simulink model "PhaseII_opalrt_NoProtection"  (Simulink 8.8)
settings: Solver=ode3  StartTime=0.0  StopTime=inf  FixedStep=Ts  RelTol=1e-5  EnableMultiTasking=on
model workspace (MAT data in the model file):
  Swing_theta = [0 -120 120]
  Swing_v = [1 1 1]
  ft2km = 0.0003048
  miperkm = 0.621371
  w = 376.991118431
  x = 0.5
  x_1 = 10
  x_2 = 1
  x_3 = 1
  x_4 = 1
  x_5 = 1
  x_6 = 1
  x_7 = 1
  x_8 : num (value not decoded)
PostLoadFcn:
  | %BESS ctrl
  | Kpf=0.005*3*12;
  | Kif=5*6;
  | 
  | Kpf1=0.005*3*12;
  | Kif1=5*6;
  | Kp_v=0.016*15*35;
  | Ki_v=12*25;
  | 
  | Kp_v1=0.016*15*35;
  | Ki_v1=12*25;
  | 
  | Vabc_B=12.47e3;
  | Vdc_ref=Vabc_B*2;
  | Kpwm=sqrt(2)*Vabc_B/Vdc_ref;
  | ZB=Vabc_B^2/1e6;
  | R=0.005*ZB;
  | Ibasefull=673/2*sqrt(2);
  | 
  | 
  | Ts_Control=1e-4;
  | ts=0.05;
  | delay=0.2;
  | offset=10e3;
  | t_plan=60;
  | t_monitor=.2;
  | t_mon=t_monitor;
  | scalingfactor=1;
  | x=0.5;
  | n=6;
  | %t_plan=1/15;
  | %t_monitor=10/900;
  | %t_mon=10/900;
  | 
  | %t_plan=1/5;
  | %t_monitor=10/300;
  | %t_mon=10/300;
  | %scalingfactor=1/300;
  | 
  | f0=60;
  | 
  | Pabc_B=1e6;
  | Iabc_B=Pabc_B*sqrt(2/3)/Vabc_B;  % pk value
  | Imax_1=2.5;
  | Ptrans_B=Pabc_B*200;
  | 
  | Vdc_ref=Vabc_B*2;
  | 
  | ZB=Vabc_B^2/Pabc_B;
  | L=0.1*ZB/2/pi/60;
  | R=0.1*ZB;
  | C=1/(4*pi^2*(2e3)^2*L);
  | 
  | LL=0.005*ZB/2/pi/60;
  | RR=0.005*ZB;
  | 
  | RC=0.02;
  | 
  | %%% Initial SOC %%%%
  | SOC_ini_BESS1=0.5;
  | SOC_ini_BESS2=0.5;
  | SOC_ini_BESS3=0.5;
  | 
  | %%% BESS1 %%%
  | fc=200;
  | fc_abc=2e3;
  | 
  | %% Pf droop %%
  | P0_BESS1=0.0*Pabc_B;
  | w0_BESS1=2*pi*60;
  | deltaw=2*pi*0.5;
  | Pmax_BESS1=.1*10;   %% pu value
  | m0_BESS1=deltaw*.5; %deltaw/Pmax_BESS1;    %Pmax_BESS1;
  | kpp_BESS1=3;
  | kpi_BESS1=30;
  | kfp_sec_BESS1=1;
  | kfi_sec_BESS1=30*0.01;
  | Imax_BESS1=Pmax_BESS1;
  | 
  | %% QV droop %%
  | Q0_BESS1=.0*Pabc_B;
  | V0_BESS1=1.03;
  | kvp_BESS1=0.01;
  | kvi_BESS1=5;
  | Dlim=.95;
  | Qmax_BESS1=Pmax_BESS1;
  | mq_BESS1=0.05*.5; %/Qmax_BESS1;
  | kvp_sec_BESS1=1;
  | kvi_sec_BESS1=5*0.05;
  | 
  | %%% BESS2 %%%
  | 
  | %% Pf droop %%
  | P0_BESS2=P0_BESS1;
  | w0_BESS2=2*pi*60;
  | deltaw=2*pi*0.5;
  | Pmax_BESS2=.1*20;   %% pu value
  | m0_BESS2=m0_BESS1;   %/Pmax_BESS2;
  | kpp_BESS2=3;
  | kpi_BESS2=30;
  | Imax_BESS2=Pmax_BESS2;
  | 
  | %% QV droop %%
  | Q0_BESS2=Q0_BESS1;
  | V0_BESS2=V0_BESS1;
  | kvp_BESS2=0.01;
  | kvi_BESS2=5;
  | Qmax_BESS2=Pmax_BESS2;
  | mq_BESS2=mq_BESS1;   %/Qmax_BESS2;
  | 
  | %%% BESS3 %%%
  | 
  | %% Pf droop %%
  | P0_BESS3=0.0*Pabc_B;
  | w0_BESS3=2*pi*60;
  | deltaw=2*pi*0.5;
  | Pmax_BESS3=.1*6;   %% pu value
  | m0_BESS3=deltaw*.5; %deltaw/Pmax_BESS3;    %Pmax_BESS1;
  | kpp_BESS3=3;
  | kpi_BESS3=30;
  | kfp_sec_BESS3=1;
  | kfi_sec_BESS3=30*0.01;
  | Imax_BESS3=Pmax_BESS3;
  | 
  | %% QV droop %%
  | Q0_BESS3=.0*Pabc_B;
  | V0_BESS3=1.03;
  | kvp_BESS3=0.01;
  | kvi_BESS3=5;
  | Dlim=.95;
  | Qmax_BESS3=Pmax_BESS3;
  | mq_BESS3=0.05*.5; %/Qmax_BESS3;
  | kvp_sec_BESS3=1;
  | kvi_sec_BESS3=5*0.05;
  | 
  | 
  | %% Outer voltage and inner current loops %%%
  | %Kp_v=0.19*0.036*20;
  | %Ki_v=0.19*5;
  | 
  | % Kp_I=2.773*0.0013/10/1.5;
  | % Ki_I =2.773/5/1.5;
  | Kp_I=2.773*0.0013; %ma /2phil 0413 /2
  | Ki_I =2.773/2/1.5; %ma /2phil 0413 /2
  | 
  | 
  | % Kp_I_PV=2.773*0.0013/2/500;
  | % Ki_I_PV =2.773/1/20000;
  | % Kp_I_PV=2.773*0.0013/10/1.5;
  | % Ki_I_PV =2.773/5/1.5;
  | Kp_I_PV=2.773*0.0013/4; %ma /2phil 0413 /2
  | Ki_I_PV =2.773/2/1.5/4; %ma /2phil 0413 /2
  | 
  | %%% single voltage loop %%%
  | Kp_vd=0.053*0.0042*0.02;
  | Ki_vd=0.053*0.02;
  | 
  | Kp_vd_neg=0.053*0.0042*0.1;
  | Ki_vd_neg=0.053*0.1;
  | 
  | coupling_pu=w0_BESS1*L/ZB*Vabc_B/Vdc_ref*1.414;%*sqrt(2)
  | 
  | 
  | %%% Load %%%
  | 
  | %% Critical Load %%
  | Pref_CL1=-161e3;
  | Qref_CL1=-50e3*0;
  | 
  | Pref_CL2=-161e3;
  | Qref_CL2=-50e3*0;
  | 
  | %% Non-critical load %%
  | Pref_NCL=-505e3*1;
  | Qref_NCL=-50e3*0;
  | 
  | %%% PV %%%
  | Qref_PV1=100e3*0;
  | Qref_PV2=100e3*0;
  | 
  | %%% BESS1 %%%
  | Pref_BESS1=100e3;
  | Qref_BESS1=100e3;
  | 
  | %%% BESS2 %%%
  | Pref_BESS2=500e3;
  | Qref_BESS2=500e3;
  | 
  | %%% Islanded detection %%%%
  | kneg=0.01;
  | Vneg_trip=0.04;
  | Nhit=50;
  | Kp_I_neg=2.773*0.0013/8;
  | Ki_I_neg =2.773/8;
  | 
  | %%% Resynchronization %%%%
  | kp_theta_BESS1=kpp_BESS1*3*10;
  | ki_theta_BESS1=kpi_BESS1*1*10;
  | kp_theta_BESS2=kp_theta_BESS1;
  | ki_theta_BESS2=ki_theta_BESS1;
  | 
  | kvp_resyn_BESS1=kvp_BESS1*3;
  | kvi_resyn_BESS1=kvi_BESS1*3;
  | kvp_resyn_BESS2=kvp_resyn_BESS1;
  | kvi_resyn_BESS2=kvi_resyn_BESS1;
  | 
  | %%% Virtual Impedance %%%%
  | L_vir=4.6685e-3;
  | R_vir=0;
  | 
  | %% harmonic compensation %%%%
  | Smax_BESS1=0.5;
  | Smax_BESS2=0.5;
  | Rvir_BESS1=-1*1;
  | Rvir_BESS2=Rvir_BESS1/1.5;
  | Lvir_BESS1=-40e-3;
  | Lvir_BESS2=Lvir_BESS1/1.5;
  | 
  | t_resyn=.25*10;
  | topen=.45*10;
  | tfault=20;
  | t_run=0.15*10;
  | Imax_BESS3_ini=3;
  | 
  | td_trans=1*1/f0;
  | td_comm=10e-3*1; Ts = 1e-4;
  | 
  | PV_0 = [0,0,0,0,0,0,0,0,0,0,0,0,0,0,0,0,0,0,0,0,0,0,0,0.00637590701003014,0.0597883305113194,0.191640198758314,0.258183655928258,0.318938480096502,0.451835046830676,0.659184087530387,0.827159209540989,1.02022332643508,1.18871489543793,1.35005293581671,1.44694872050258,1.52351715157350,1.70617264822951,1.84211772778079,1.88159346030552,1.92819173463478,1.95215782620083,1.94381351836891,2,1.97817052341903,1.98389128053032,1.95943530210305,1.90454584020392,1.83270216133066,1.74331256478643,1.68711132752699,1.64586049291177,1.53600483984610,1.40476385461279,1.29483442340538,1.11929409073974,0.908933426293792,0.676474732830904,0.512353780945319,0.359824850691486,0.238560145785608,0.135084826418477,0.0524857700409100,0.00608374556870036,0,0,0,0,0,0,0,0,0,0,0,0,0,0,0,0,0,0,0,0,0,0,0,0,0,0,0,0,0,0];
  | BESS_limit=1.5;
  | 
  | 
  | B_OL = [6.9443e-06 2.8805e-06];
  | B_UG = [6.00927e-05 3.73399e-05];
  | Omega = 376.9911184307752;
  | R_OL = [0.17 0.527];
  | R_UG = [0.1853 0.8313];
  | X_OL = [0.6283 2.0185];
  | X_UG = [0.3144 0.3404];
  | ft2km = 0.0003048;
  | load_scale = 0.5;
  | 
  | 
  | wb = 2*pi*60; %frequency of input voltage
  | Vb = 12.47e3*sqrt(2/3); % phase voltage amplitude
  | Pb = 1e6; % Pb=2.552kW
  | Ib = Pb/(3/2*Vb); %pha
  | %%generator electrical parameters, stator resistance ignored
  | xd=3.4375;
  | xq=1.7499;
  | xdp=0.2626;
  | xqp=0.1790;
  | Td0p=2.389;
  | Tq0p=0.07;
  | 
  | %%excitation
  | KA=200;
  | TA=0.01;
  | Efdmin=-4.5; %% field voltage lower limit
  | Efdmax=4.5; %% field voltage upper limit
  | 
  | %%inertia
  | H1=7;%6.5;
  | H2=10;%6.175;
  | D=2;
  | M1=2*H1;
  | M2=2*H2;
  | 
  | %%AGC parameters (different parameters in the simulation; AGC integrates every 2 seconds, disabled before 70s)
  | B1=41; %%in simulation B1=21
  | KI=0.8; %%in simulation KI=0.05
  | 
  | %%droop
  | R_1=20;
  | 
  | %%governor
  | TG=0.2;
  | 
  | %%turbine
  | FHP=0.3;
  | TRH=7.0;
  | TCH=0.3;
  | 
  | Ts=8e-5;
InitFcn:
  | %BESS ctrl
  | Kpf=0.005*3*12;
  | Kif=5*6;
  | 
  | Kpf1=0.005*3*12;
  | Kif1=5*6;
  | Kp_v=0.016*15*35;
  | Ki_v=12*25;
  | 
  | Kp_v1=0.016*15*35;
  | Ki_v1=12*25;
  | 
  | Vabc_B=12.47e3;
  | Vdc_ref=Vabc_B*2;
  | Kpwm=sqrt(2)*Vabc_B/Vdc_ref;
  | ZB=Vabc_B^2/1e6;
  | R=0.005*ZB;
  | Ibasefull=673/2*sqrt(2);
  | 
  | 
  | Ts_Control=1e-4;
  | ts=0.05;
  | delay=0.2;
  | offset=10e3;
  | t_plan=60;
  | t_monitor=.2;
  | t_mon=t_monitor;
  | scalingfactor=1;
  | x=0.5;
  | n=6;
  | %t_plan=1/15;
  | %t_monitor=10/900;
  | %t_mon=10/900;
  | 
  | %t_plan=1/5;
  | %t_monitor=10/300;
  | %t_mon=10/300;
  | %scalingfactor=1/300;
  | 
  | f0=60;
  | 
  | Pabc_B=1e6;
  | Iabc_B=Pabc_B*sqrt(2/3)/Vabc_B;  % pk value
  | Imax_1=2.5;
  | Ptrans_B=Pabc_B*200;
  | 
  | Vdc_ref=Vabc_B*2;
  | 
  | ZB=Vabc_B^2/Pabc_B;
  | L=0.1*ZB/2/pi/60;
  | R=0.1*ZB;
  | C=1/(4*pi^2*(2e3)^2*L);
  | 
  | LL=0.005*ZB/2/pi/60;
  | RR=0.005*ZB;
  | 
  | RC=0.02;
  | 
  | %%% Initial SOC %%%%
  | SOC_ini_BESS1=0.5;
  | SOC_ini_BESS2=0.5;
  | SOC_ini_BESS3=0.5;
  | 
  | %%% BESS1 %%%
  | fc=200;
  | fc_abc=2e3;
  | 
  | %% Pf droop %%
  | P0_BESS1=0.0*Pabc_B;
  | w0_BESS1=2*pi*60;
  | deltaw=2*pi*0.5;
  | Pmax_BESS1=.1*10;   %% pu value
  | m0_BESS1=deltaw*.5; %deltaw/Pmax_BESS1;    %Pmax_BESS1;
  | kpp_BESS1=3;
  | kpi_BESS1=30;
  | kfp_sec_BESS1=1;
  | kfi_sec_BESS1=30*0.01;
  | Imax_BESS1=Pmax_BESS1;
  | 
  | %% QV droop %%
  | Q0_BESS1=.0*Pabc_B;
  | V0_BESS1=1.03;
  | kvp_BESS1=0.01;
  | kvi_BESS1=5;
  | Dlim=.95;
  | Qmax_BESS1=Pmax_BESS1;
  | mq_BESS1=0.05*.5; %/Qmax_BESS1;
  | kvp_sec_BESS1=1;
  | kvi_sec_BESS1=5*0.05;
  | 
  | %%% BESS2 %%%
  | 
  | %% Pf droop %%
  | P0_BESS2=P0_BESS1;
  | w0_BESS2=2*pi*60;
  | deltaw=2*pi*0.5;
  | Pmax_BESS2=.1*20;   %% pu value
  | m0_BESS2=m0_BESS1;   %/Pmax_BESS2;
  | kpp_BESS2=3;
  | kpi_BESS2=30;
  | Imax_BESS2=Pmax_BESS2;
  | 
  | %% QV droop %%
  | Q0_BESS2=Q0_BESS1;
  | V0_BESS2=V0_BESS1;
  | kvp_BESS2=0.01;
  | kvi_BESS2=5;
  | Qmax_BESS2=Pmax_BESS2;
  | mq_BESS2=mq_BESS1;   %/Qmax_BESS2;
  | 
  | %%% BESS3 %%%
  | 
  | %% Pf droop %%
  | P0_BESS3=0.0*Pabc_B;
  | w0_BESS3=2*pi*60;
  | deltaw=2*pi*0.5;
  | Pmax_BESS3=.1*6;   %% pu value
  | m0_BESS3=deltaw*.5; %deltaw/Pmax_BESS3;    %Pmax_BESS1;
  | kpp_BESS3=3;
  | kpi_BESS3=30;
  | kfp_sec_BESS3=1;
  | kfi_sec_BESS3=30*0.01;
  | Imax_BESS3=Pmax_BESS3;
  | 
  | %% QV droop %%
  | Q0_BESS3=.0*Pabc_B;
  | V0_BESS3=1.03;
  | kvp_BESS3=0.01;
  | kvi_BESS3=5;
  | Dlim=.95;
  | Qmax_BESS3=Pmax_BESS3;
  | mq_BESS3=0.05*.5; %/Qmax_BESS3;
  | kvp_sec_BESS3=1;
  | kvi_sec_BESS3=5*0.05;
  | 
  | 
  | %% Outer voltage and inner current loops %%%
  | %Kp_v=0.19*0.036*20;
  | %Ki_v=0.19*5;
  | 
  | % Kp_I=2.773*0.0013/10/1.5;
  | % Ki_I =2.773/5/1.5;
  | Kp_I=2.773*0.0013; %ma /2phil 0413 /2
  | Ki_I =2.773/2/1.5; %ma /2phil 0413 /2
  | 
  | 
  | % Kp_I_PV=2.773*0.0013/2/500;
  | % Ki_I_PV =2.773/1/20000;
  | % Kp_I_PV=2.773*0.0013/10/1.5;
  | % Ki_I_PV =2.773/5/1.5;
  | Kp_I_PV=2.773*0.0013/4; %ma /2phil 0413 /2
  | Ki_I_PV =2.773/2/1.5/4; %ma /2phil 0413 /2
  | 
  | %%% single voltage loop %%%
  | Kp_vd=0.053*0.0042*0.02;
  | Ki_vd=0.053*0.02;
  | 
  | Kp_vd_neg=0.053*0.0042*0.1;
  | Ki_vd_neg=0.053*0.1;
  | 
  | coupling_pu=w0_BESS1*L/ZB*Vabc_B/Vdc_ref*1.414;%*sqrt(2)
  | 
  | 
  | %%% Load %%%
  | 
  | %% Critical Load %%
  | Pref_CL1=-161e3;
  | Qref_CL1=-50e3*0;
  | 
  | Pref_CL2=-161e3;
  | Qref_CL2=-50e3*0;
  | 
  | %% Non-critical load %%
  | Pref_NCL=-505e3*1;
  | Qref_NCL=-50e3*0;
  | 
  | %%% PV %%%
  | Qref_PV1=100e3*0;
  | Qref_PV2=100e3*0;
  | 
  | %%% BESS1 %%%
  | Pref_BESS1=100e3;
  | Qref_BESS1=100e3;
  | 
  | %%% BESS2 %%%
  | Pref_BESS2=500e3;
  | Qref_BESS2=500e3;
  | 
  | %%% Islanded detection %%%%
  | kneg=0.01;
  | Vneg_trip=0.04;
  | Nhit=50;
  | Kp_I_neg=2.773*0.0013/8;
  | Ki_I_neg =2.773/8;
  | 
  | %%% Resynchronization %%%%
  | kp_theta_BESS1=kpp_BESS1*3*10;
  | ki_theta_BESS1=kpi_BESS1*1*10;
  | kp_theta_BESS2=kp_theta_BESS1;
  | ki_theta_BESS2=ki_theta_BESS1;
  | 
  | kvp_resyn_BESS1=kvp_BESS1*3;
  | kvi_resyn_BESS1=kvi_BESS1*3;
  | kvp_resyn_BESS2=kvp_resyn_BESS1;
  | kvi_resyn_BESS2=kvi_resyn_BESS1;
  | 
  | %%% Virtual Impedance %%%%
  | L_vir=4.6685e-3;
  | R_vir=0;
  | 
  | %% harmonic compensation %%%%
  | Smax_BESS1=0.5;
  | Smax_BESS2=0.5;
  | Rvir_BESS1=-1*1;
  | Rvir_BESS2=Rvir_BESS1/1.5;
  | Lvir_BESS1=-40e-3;
  | Lvir_BESS2=Lvir_BESS1/1.5;
  | 
  | t_resyn=.25*10;
  | topen=.45*10;
  | tfault=20;
  | t_run=0.15*10;
  | Imax_BESS3_ini=3;
  | 
  | td_trans=1*1/f0;
  | td_comm=10e-3*1; Ts = 1e-4;
  | 
  | PV_0 = [0,0,0,0,0,0,0,0,0,0,0,0,0,0,0,0,0,0,0,0,0,0,0,0.00637590701003014,0.0597883305113194,0.191640198758314,0.258183655928258,0.318938480096502,0.451835046830676,0.659184087530387,0.827159209540989,1.02022332643508,1.18871489543793,1.35005293581671,1.44694872050258,1.52351715157350,1.70617264822951,1.84211772778079,1.88159346030552,1.92819173463478,1.95215782620083,1.94381351836891,2,1.97817052341903,1.98389128053032,1.95943530210305,1.90454584020392,1.83270216133066,1.74331256478643,1.68711132752699,1.64586049291177,1.53600483984610,1.40476385461279,1.29483442340538,1.11929409073974,0.908933426293792,0.676474732830904,0.512353780945319,0.359824850691486,0.238560145785608,0.135084826418477,0.0524857700409100,0.00608374556870036,0,0,0,0,0,0,0,0,0,0,0,0,0,0,0,0,0,0,0,0,0,0,0,0,0,0,0,0,0,0];
  | BESS_limit=1.5;
  | 
  | 
  | B_OL = [6.9443e-06 2.8805e-06];
  | B_UG = [6.00927e-05 3.73399e-05];
  | Omega = 376.9911184307752;
  | R_OL = [0.17 0.527];
  | R_UG = [0.1853 0.8313];
  | X_OL = [0.6283 2.0185];
  | X_UG = [0.3144 0.3404];
  | ft2km = 0.0003048;
  | load_scale = 0.5;
  | 
  | 
  | wb = 2*pi*60; %frequency of input voltage
  | Vb = 12.47e3*sqrt(2/3); % phase voltage amplitude
  | Pb = 1e6; % Pb=2.552kW
  | Ib = Pb/(3/2*Vb); %pha
  | %%generator electrical parameters, stator resistance ignored
  | xd=3.4375;
  | xq=1.7499;
  | xdp=0.2626;
  | xqp=0.1790;
  | Td0p=2.389;
  | Tq0p=0.07;
  | 
  | %%excitation
  | KA=200;
  | TA=0.01;
  | Efdmin=-4.5; %% field voltage lower limit
  | Efdmax=4.5; %% field voltage upper limit
  | 
  | %%inertia
  | H1=7;%6.5;
  | H2=10;%6.175;
  | D=2;
  | M1=2*H1;
  | M2=2*H2;
  | 
  | %%AGC parameters (different parameters in the simulation; AGC integrates every 2 seconds, disabled before 70s)
  | B1=41; %%in simulation B1=21
  | KI=0.8; %%in simulation KI=0.05
  | 
  | %%droop
  | R_1=20;
  | 
  | %%governor
  | TG=0.2;
  | 
  | %%turbine
  | FHP=0.3;
  | TRH=7.0;
  | TCH=0.3;
  | 
  | Ts=8e-5;
undefined symbols (not defined in the file): D1, Delta, DiscIntNeverNeededParam, Left, PG2ref, type, V
libraries: powerlib x220, powerlib_meascontrol x82, dspstat3 x54, dsparch4 x43, dspswit3 x24, simulink x19, simulink_extras x12, powerlib_extras x11, ssn_lib x7, artemis x6, rtlab x5, rtio_generic_dnp3 x5
(part 1 of 9)
settings Model: ARTEMISmethode_block_infos=$$__separator__$$PhaseII_opalrt_NoProtection/ARTEMIS Guide$$__separator__$$  Creator=AmineYamane  LastModifiedBy=iray1
settings OptimizationCC: BlockReduction=off  BooleanDataType=off  OptimizeBlockIOStorage=off  BufferReuse=off  GlobalBufferReuse=off  ExpressionFolding=off  ExpressionDepthLimit=2147483647  LocalBlockOutputs=off
settings DebuggingCC: SolverPrmCheckMsg=warning  MultiTaskCondExecSysMsg=warning  UnconnectedInputMsg=none  UnconnectedOutputMsg=none  UnconnectedLineMsg=none
settings ModelReferenceCC: ModelReferenceMinAlgLoopOccurrences=on
settings ConfigComp: CovSFcnEnable=off

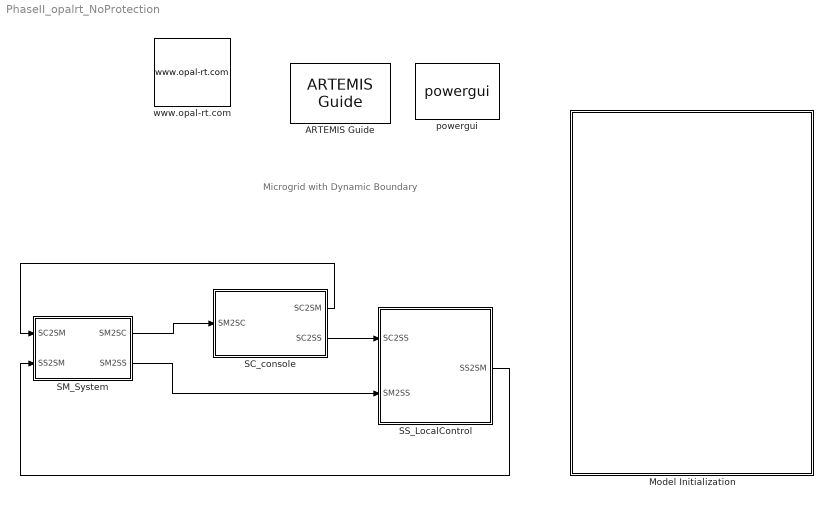
== system PhaseII_opalrt_NoProtection ==
  note: Microgrid with Dynamic Boundary
  ARTEMIS Guide : artemis/ARTEMIS/ARTEMIS Guide  Tag=FTSSmethode_opal_4hx0r99  Description=5.0_z1  lock=on  Ts=Ts  opt=art5  dyna=off  nb_perm=50  RT_fullcomp=off  ssn=on  ssn_itvc=off  ssn_ivic=off  ssn_ext=off  ssn_solver=Backward Euler  ssn_impulse=off  ssn_quasimpulse=off  ssn_impulse_loop=2  paraExtinctionThy=off  Thy_Impulse=on  dtc=Off  dtc_opt=true impulse event detection  ao=on  simtype=off  ct_mac=off  lin_mov=off  lsp=[0.001 2]  spike_skip=Disabled  dtc_extra=1  dtc_sws=normal  dtc_pied=0.5  SPSRulesBlock=SPSRules  tre=on  ctmm=off  LF=off  dpl_type=ARTEMiS DPL  rlc_type=off  custom_type=off  para=off  ssn_ImpulseLoopBlockedStateUpdate=2  ssn_mov_iter_number=5  ssn_switch_iter_number=5  ssn_nib_type_verify=on  ssn_use_lu=on  ssn_use_ldlt=off
  Model Initialization : Subsystem  mask(Model Functions){InitFcnX=|, prel=off, posl=on, inif=on, strf=off}
      mask InitFcnX=|
      | %BESS ctrl
      | Kpf=0.005*3*12;
      | Kif=5*6;
      |
      | Kpf1=0.005*3*12;
      | Kif1=5*6;
      | Kp_v=0.016*15*35;
      | Ki_v=12*25;
      |
      | Kp_v1=0.016*15*35;
      | Ki_v1=12*25;
      |
      | Vabc_B=12.47e3;
      | Vdc_ref=Vabc_B*2;
      | Kpwm=sqrt(2)*Vabc_B/Vdc_ref;
      | ZB=Vabc_B^2/1e6;
      | R=0.005*ZB;
      | Ibasefull=673/2*sqrt(2);
      |
      |
      | Ts_Control=1e-4;
      | ts=0.05;
      | delay=0.2;
      | offset=10e3;
      | t_plan=60;
      | t_monitor=.2;
      | t_mon=t_monitor;
      | scalingfactor=1;
      | x=0.5;
      | n=6;
      | %t_plan=1/15;
      | %t_monitor=10/900;
      | %t_mon=10/900;
      |
      | %t_plan=1/5;
      | %t_monitor=10/300;
      | %t_mon=10/300;
      | %scalingfactor=1/300;
      |
      | f0=60;
      |
      | Pabc_B=1e6;
      | Iabc_B=Pabc_B*sqrt(2/3)/Vabc_B;  % pk value
      | Imax_1=2.5;
      | Ptrans_B=Pabc_B*200;
      |
      | Vdc_ref=Vabc_B*2;
      |
      | ZB=Vabc_B^2/Pabc_B;
      | L=0.1*ZB/2/pi/60;
      | R=0.1*ZB;
      | C=1/(4*pi^2*(2e3)^2*L);
      |
      | LL=0.005*ZB/2/pi/60;
      | RR=0.005*ZB;
      |
      | RC=0.02;
      |
      | %%% Initial SOC %%%%
      | SOC_ini_BESS1=0.5;
      | SOC_ini_BESS2=0.5;
      | SOC_ini_BESS3=0.5;
      |
      | %%% BESS1 %%%
      | fc=200;
      | fc_abc=2e3;
      |
      | %% Pf droop %%
      | P0_BESS1=0.0*Pabc_B;
      | w0_BESS1=2*pi*60;
      | deltaw=2*pi*0.5;
      | Pmax_BESS1=.1*10;   %% pu value
      | m0_BESS1=deltaw*.5; %deltaw/Pmax_BESS1;    %Pmax_BESS1;
      | kpp_BESS1=3;
      | kpi_BESS1=30;
      | kfp_sec_BESS1=1;
      | kfi_sec_BESS1=30*0.01;
      | Imax_BESS1=Pmax_BESS1;
      |
      | %% QV droop %%
      | Q0_BESS1=.0*Pabc_B;
      | V0_BESS1=1.03;
      | kvp_BESS1=0.01;
      | kvi_BESS1=5;
      | Dlim=.95;
      | Qmax_BESS1=Pmax_BESS1;
      | mq_BESS1=0.05*.5; %/Qmax_BESS1;
      | kvp_sec_BESS1=1;
      | kvi_sec_BESS1=5*0.05;
      |
      | %%% BESS2 %%%
      |
      | %% Pf droop %%
      | P0_BESS2=P0_BESS1;
      | w0_BESS2=2*pi*60;
      | deltaw=2*pi*0.5;
      | Pmax_BESS2=.1*20;   %% pu value
      | m0_BESS2=m0_BESS1;   %/Pmax_BESS2;
      | kpp_BESS2=3;
      | kpi_BESS2=30;
      | Imax_BESS2=Pmax_BESS2;
      |
      | %% QV droop %%
      | Q0_BESS2=Q0_BESS1;
      | V0_BESS2=V0_BESS1;
      | kvp_BESS2=0.01;
      | kvi_BESS2=5;
      | Qmax_BESS2=Pmax_BESS2;
      | mq_BESS2=mq_BESS1;   %/Qmax_BESS2;
      |
      | %%% BESS3 %%%
      |
      | %% Pf droop %%
      | P0_BESS3=0.0*Pabc_B;
      | w0_BESS3=2*pi*60;
      | deltaw=2*pi*0.5;
      | Pmax_BESS3=.1*6;   %% pu value
      | m0_BESS3=deltaw*.5; %deltaw/Pmax_BESS3;    %Pmax_BESS1;
      | kpp_BESS3=3;
      | kpi_BESS3=30;
      | kfp_sec_BESS3=1;
      | kfi_sec_BESS3=30*0.01;
      | Imax_BESS3=Pmax_BESS3;
      |
      | %% QV droop %%
      | Q0_BESS3=.0*Pabc_B;
      | V0_BESS3=1.03;
      | kvp_BESS3=0.01;
      | kvi_BESS3=5;
      | Dlim=.95;
      | Qmax_BESS3=Pmax_BESS3;
      | mq_BESS3=0.05*.5; %/Qmax_BESS3;
      | kvp_sec_BESS3=1;
      | kvi_sec_BESS3=5*0.05;
      |
      |
      | %% Outer voltage and inner current loops %%%
      | %Kp_v=0.19*0.036*20;
      | %Ki_v=0.19*5;
      |
      | % Kp_I=2.773*0.0013/10/1.5;
      | % Ki_I =2.773/5/1.5;
      | Kp_I=2.773*0.0013; %ma /2phil 0413 /2
      | Ki_I =2.773/2/1.5; %ma /2phil 0413 /2
      |
      |
      | % Kp_I_PV=2.773*0.0013/2/500;
      | % Ki_I_PV =2.773/1/20000;
      | % Kp_I_PV=2.773*0.0013/10/1.5;
      | % Ki_I_PV =2.773/5/1.5;
      | Kp_I_PV=2.773*0.0013/4; %ma /2phil 0413 /2
      | Ki_I_PV =2.773/2/1.5/4; %ma /2phil 0413 /2
      |
      | %%% single voltage loop %%%
      | Kp_vd=0.053*0.0042*0.02;
      | Ki_vd=0.053*0.02;
      |
      | Kp_vd_neg=0.053*0.0042*0.1;
      | Ki_vd_neg=0.053*0.1;
      |
      | coupling_pu=w0_BESS1*L/ZB*Vabc_B/Vdc_ref*1.414;%*sqrt(2)
      |
      |
      | %%% Load %%%
      |
      | %% Critical Load %%
      | Pref_CL1=-161e3;
      | Qref_CL1=-50e3*0;
      |
      | Pref_CL2=-161e3;
      | Qref_CL2=-50e3*0;
      |
      | %% Non-critical load %%
      | Pref_NCL=-505e3*1;
      | Qref_NCL=-50e3*0;
      |
      | %%% PV %%%
      | Qref_PV1=100e3*0;
      | Qref_PV2=100e3*0;
      |
      | %%% BESS1 %%%
      | Pref_BESS1=100e3;
      | Qref_BESS1=100e3;
      |
      | %%% BESS2 %%%
      | Pref_BESS2=500e3;
      | Qref_BESS2=500e3;
      |
      | %%% Islanded detection %%%%
      | kneg=0.01;
      | Vneg_trip=0.04;
      | Nhit=50;
      | Kp_I_neg=2.773*0.0013/8;
      | Ki_I_neg =2.773/8;
      |
      | %%% Resynchronization %%%%
      | kp_theta_BESS1=kpp_BESS1*3*10;
      | ki_theta_BESS1=kpi_BESS1*1*10;
      | kp_theta_BESS2=kp_theta_BESS1;
      | ki_theta_BESS2=ki_theta_BESS1;
      |
      | kvp_resyn_BESS1=kvp_BESS1*3;
      | kvi_resyn_BESS1=kvi_BESS1*3;
      | kvp_resyn_BESS2=kvp_resyn_BESS1;
      | kvi_resyn_BESS2=kvi_resyn_BESS1;
      |
      | %%% Virtual Impedance %%%%
      | L_vir=4.6685e-3;
      | R_vir=0;
      |
      | %% harmonic compensation %%%%
      | Smax_BESS1=0.5;
      | Smax_BESS2=0.5;
      | Rvir_BESS1=-1*1;
      | Rvir_BESS2=Rvir_BESS1/1.5;
      | Lvir_BESS1=-40e-3;
      | Lvir_BESS2=Lvir_BESS1/1.5;
      |
      | t_resyn=.25*10;
      | topen=.45*10;
      | tfault=20;
      | t_run=0.15*10;
      | Imax_BESS3_ini=3;
      |
      | td_trans=1*1/f0;
      | td_comm=10e-3*1; Ts = 1e-4;
      |
      | PV_0 = [0,0,0,0,0,0,0,0,0,0,0,0,0,0,0,0,0,0,0,0,0,0,0,0.00637590701003014,0.0597883305113194,0.191640198758314,0.258183655928258,0.318938480096502,0.451835046830676,0.659184087530387,0.827159209540989,1.02022332643508,1.18871489543793,1.35005293581671,1.44694872050258,1.52351715157350,1.70617264822951,1.84211772778079,1.88159346030552,1.92819173463478,1.95215782620083,1.94381351836891,2,1.97817052341903,1.98389128053032,1.95943530210305,1.90454584020392,1.83270216133066,1.74331256478643,1.68711132752699,1.64586049291177,1.53600483984610,1.40476385461279,1.29483442340538,1.11929409073974,0.908933426293792,0.676474732830904,0.512353780945319,0.359824850691486,0.238560145785608,0.135084826418477,0.0524857700409100,0.00608374556870036,0,0,0,0,0,0,0,0,0,0,0,0,0,0,0,0,0,0,0,0,0,0,0,0,0,0,0,0,0,0];
      | BESS_limit=1.5;
      |
      |
      | B_OL = [6.9443e-06 2.8805e-06];
      | B_UG = [6.00927e-05 3.73399e-05];
      | Omega = 376.9911184307752;
      | R_OL = [0.17 0.527];
      | R_UG = [0.1853 0.8313];
      | X_OL = [0.6283 2.0185];
      | X_UG = [0.3144 0.3404];
      | ft2km = 0.0003048;
      | load_scale = 0.5;
      |
      |
      | wb = 2*pi*60; %frequency of input voltage
      | Vb = 12.47e3*sqrt(2/3); % phase voltage amplitude
      | Pb = 1e6; % Pb=2.552kW
      | Ib = Pb/(3/2*Vb); %pha
      | %%generator electrical parameters, stator resistance ignored
      | xd=3.4375;
      | xq=1.7499;
      | xdp=0.2626;
      | xqp=0.1790;
      | Td0p=2.389;
      | Tq0p=0.07;
      |
      | %%excitation
      | KA=200;
      | TA=0.01;
      | Efdmin=-4.5; %% field voltage lower limit
      | Efdmax=4.5; %% field voltage upper limit
      |
      | %%inertia
      | H1=7;%6.5;
      | H2=10;%6.175;
      | D=2;
      | M1=2*H1;
      | M2=2*H2;
      |
      | %%AGC parameters (different parameters in the simulation; AGC integrates every 2 seconds, disabled before 70s)
      | B1=41; %%in simulation B1=21
      | KI=0.8; %%in simulation KI=0.05
      |
      | %%droop
      | R_1=20;
      |
      | %%governor
      | TG=0.2;
      |
      | %%turbine
      | FHP=0.3;
      | TRH=7.0;
      | TCH=0.3;
      |
      | Ts=8e-5;
      mask prompts: InitFcnX "Initialisation"; prel "Preload Function"; posl "PostLoad Function"; inif "InitFcn"; strf "StartFcn"
      mask init:
      | currentBlock = gcb;
      | root = bdroot(currentBlock);
      | 
      | if ~strcmp(get_param(root,'BlockDiagramType'),'library')
      |     if prel==1
      |         set_param(root, 'PreLoadFcn', InitFcnX);
      |     else
      |         set_param(root, 'PreLoadFcn', '');
      |     end
      |     if inif==1
      |         set_param(root, 'InitFcn', InitFcnX);
      |     else
      |         set_param(root, 'InitFcn', '');
      |     end
      |     if strf==1
      |         set_param(root, 'StartFcn', InitFcnX);
      |     else
      |         set_param(root, 'StartFcn', '');
      |     end
      |     if posl==1
      |         set_param(root, 'PostLoadFcn', InitFcnX);
      |     else
      |         set_param(root, 'PostLoadFcn', '');
      |     end
      | end
      | 
      | pos = get_param(currentBlock, 'Position');
      | width = pos(3) - pos(1); height = pos(4) - pos(2);
      | txt = [ upper(root) '\n' '- InitFcn. . . . . '  get_param(root, 'InitFcn') ];
      settings: CopyFcn=set_param(gcb,'LinkStatus','none')
      mask Display: text(5, height*0.5, txt, 'horizontalAlignment', 'left', 'verticalAlignment', 'middle') ;
  SC_console : Subsystem
  SM_System : Subsystem
  SS_LocalControl : Subsystem
  powergui : powerlib/powergui  Priority=1  SimulationMode=Discrete  SolverType=Tustin  SampleTime=Ts  frequency=60  SPID=off  DisableSnubberDevices=off  DisableRonSwitches=off  DisableVfSwitches=off  SwTol=0  DisplayEquations=off  Interpol=off  ExternalGateDelay=off  methode=off  Ts=0  FunctionMessages=off  echomessages=off  HookPort=off  EnableUseOfTLC=off  x0status=steady  frequencyindice=0  Pbase=100e6  ErrMax=1e-4  Iterations=50  UnitsV=kV  UnitsW=MW  buscounter=0  RestoreLinks=warning  ResistiveCurrentMeasurement=off  Frange=[0:2:500]  Ylog=off  Xlog=on  ShowGrid=off  save=off  variable=ZData  structure=0  ZoomFFT=on  StartTime=0.0  cycles=1  DisplayStyle=1  fundamental=60  FreqAxis=off  MaxFrequency=1000  frequencyindicesteady=1  RmsSteady=1  display=off
  www.opal-rt.com : artemis/Internal/www.opal-rt.com  SystemSampleTime=-1
  wires:
  SC_console/1(SC2SM) -> SM_System/1(SC2SM)
  SS_LocalControl/1("SS2SM ") -> SM_System/2(SS2SM)
  SM_System/1(SM2SC) -> SC_console/1(SM2SC)
  SC_console/2(SC2SS) -> SS_LocalControl/1(SC2SS)
  SM_System/2(SM2SS) -> SS_LocalControl/2(SM2SS)

== system PhaseII_opalrt_NoProtection/Model Initialization ==

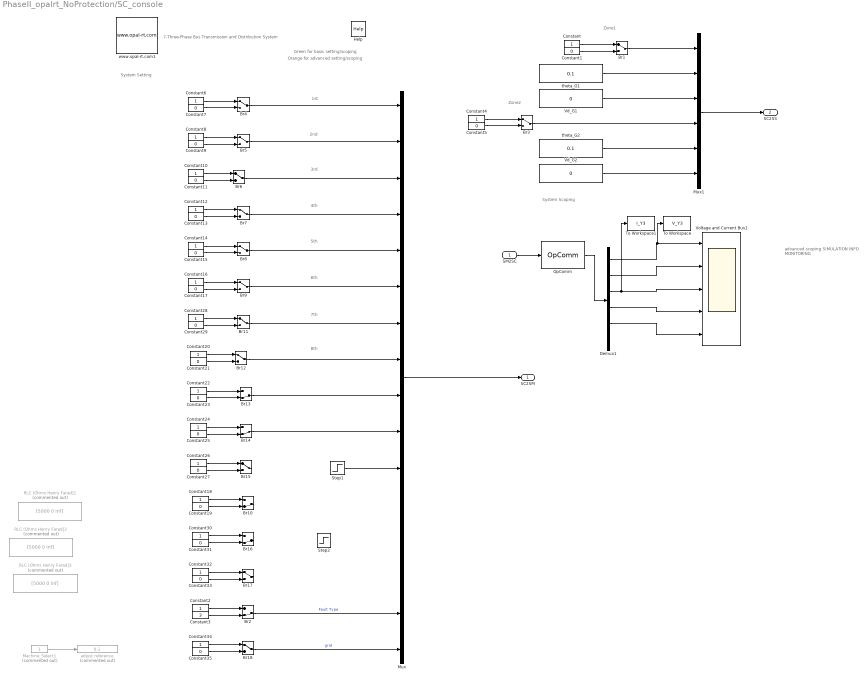
== system PhaseII_opalrt_NoProtection/SC_console ==
  note: System Setting
  note: Green for basic setting/scoping
  note: Orange for advanced setting/scoping
  note: System Scoping
  note: advanced scoping
      | SIMULATION INFO MONITORING
  note: 7-Three-Phase Bus Transmission and Distribution System
  note: Zone1
  note: Zone2
  note: 1st
  note: 2nd
  note: 3rd
  note: 4th
  note: 5th
  note: 6th
  note: 7th
  note: 8th
  SM2SC : Inport
  Br{1,3..9,11..12,15,17..18} (13 alike) : ManualSwitch
  Br{2,10,13..14,16} (5 alike) : ManualSwitch  CurrentSetting=0
  Constant{,2,4,6,8,10,12,14,16,18,20,22,24,26,28,30,32,34} (18 alike) : Constant
  Constant{1,5,7,9,11,13,15,17,19,21,23,25,27,29,31,33,35} (17 alike) : Constant  Value=0
  Constant3 : Constant  Value=3
  Demux1 : Demux  Outputs=[3 3 1 3 3 3]
  Help : artemis/Internal/Help  docfile=..\help\adgrid22_7bus_hvac.html
  Machine_Select1 : Constant  Commented=on
  Mux : Mux  Inputs=[1 1 1 1 1 1 1 1 1 1 1 1 1 1 1 1]
  Mux1 : Mux  Inputs=[1 1 1 1 1 1]
  OpComm : rtlab/OpComm  nbport=1  groupe_acq=1  subsys_rate=0  st=0  Synchronization=on  Interpolation=on  Threshold=1.0  Missed_Data=off  Sim_Time=off  Samples=off  dynSigOut=off  from_console=0  warning_done=off  writeOpCommFile=off  Offset=off
  RLC (Ohms Henry Farad]1 : Constant  Commented=on  Value=[5000 0 inf]
  RLC (Ohms Henry Farad]2 : Constant  Commented=on  Value=[5000 0 inf]
  RLC (Ohms Henry Farad]3 : Constant  Commented=on  Value=[5000 0 inf]
  Step1 : Step  Time=15  SampleTime=0
  Step2 : Step  Time=8  SampleTime=0
  To Workspace : ToWorkspace  VariableName=V_Y3  SaveFormat=Timeseries  SampleTime=-1
  To Workspace1 : ToWorkspace  VariableName=I_Y3  SaveFormat=Timeseries  SampleTime=-1
  Vd_G1 : Constant  Value=0
  Vd_G2 : Constant  Value=0
  Voltage and Current Bus1 : Scope  NumInputPorts=5
  adjust reference : simulink/Math Operations/Slider Gain  Commented=on  low=0  gain=0.1  high=1
  theta_G1 : Constant  Value=0.1
  theta_G2 : Constant  Value=0.1
  www.opal-rt.com1 : artemis/Internal/www.opal-rt.com  SystemSampleTime=-1
  SC2SM : Outport
  SC2SS : Outport  Port=2
  wires:
  SM2SC/1 -> OpComm/1
  Mux/1 -> SC2SM/1
  Constant/1 -> Br1/1
  Constant1/1 -> Br1/2
  Constant6/1 -> Br4/1
  Constant7/1 -> Br4/2
  Constant8/1 -> Br5/1
  Constant9/1 -> Br5/2
  Constant12/1 -> Br7/1
  Constant13/1 -> Br7/2
  Constant14/1 -> Br8/1
  Constant15/1 -> Br8/2
  Constant16/1 -> Br9/1
  Constant17/1 -> Br9/2
  Constant10/1 -> Br6/1
  Constant11/1 -> Br6/2
  OpComm/1 -> Demux1/1
  Constant2/1 -> Br2/1
  Constant3/1 -> Br2/2
  Machine_Select1/1 -> adjust reference/1
  Br1/1 -> Mux1/1
  Mux1/1 -> SC2SS/1
  theta_G1/1 -> Mux1/2
  Vd_G1/1 -> Mux1/3
  Constant28/1 -> Br11/1
  Constant29/1 -> Br11/2
  Constant22/1 -> Br13/1
  Constant23/1 -> Br13/2
  Constant24/1 -> Br14/1
  Constant25/1 -> Br14/2
  Constant26/1 -> Br15/1
  Constant27/1 -> Br15/2
  Constant20/1 -> Br12/1
  Constant21/1 -> Br12/2
  Br4/1 -> Mux/1
  Br5/1 -> Mux/2
  Br9/1 -> Mux/6
  Br13/1 -> Mux/9
  Br14/1 -> Mux/10
  Br2/1 -> Mux/15  "Fault Type"
  Constant4/1 -> Br3/1
  Constant5/1 -> Br3/2
  Br3/1 -> Mux1/4
  theta_G2/1 -> Mux1/5
  Vd_G2/1 -> Mux1/6
  Constant18/1 -> Br10/1
  Constant19/1 -> Br10/2
  Constant30/1 -> Br16/1
  Constant31/1 -> Br16/2
  Constant32/1 -> Br17/1
  Constant33/1 -> Br17/2
  Constant34/1 -> Br18/1
  Constant35/1 -> Br18/2
  Br18/1 -> Mux/16  "grid"
  Demux1/1 -> To Workspace/1, Voltage and Current Bus1/1
  Br6/1 -> Mux/3
  Br11/1 -> Mux/7
  Br7/1 -> Mux/4
  Br12/1 -> Mux/8
  Br8/1 -> Mux/5
  Demux1/2 -> Voltage and Current Bus1/2
  Demux1/3 -> To Workspace1/1, Voltage and Current Bus1/3
  Demux1/4 -> Voltage and Current Bus1/4
  Demux1/5 -> Voltage and Current Bus1/5
  Step1/1 -> Mux/11
